simulink model "pid_and_statefeedback"  (R2021b)
settings: Solver=VariableStepAuto  StartTime=0.0  StopTime=10.0  RelTol=1e-3
undefined symbols (not defined in the file): mA, mB, mC, mD, mK, mL
libraries: slpidlib x1, simulink x1
settings Model: Creator=insha  LastModifiedBy=insha

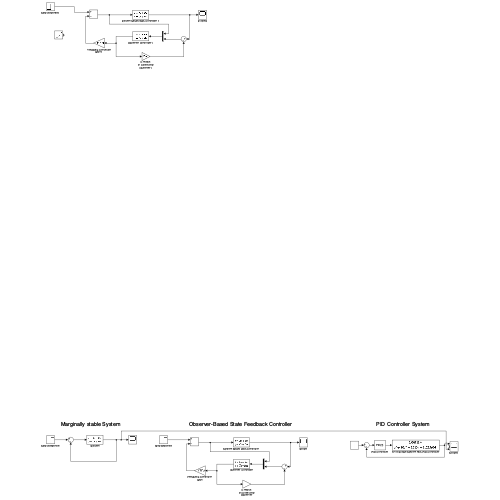
[thumbnail: Simulink's stored preview of the top-level diagram]
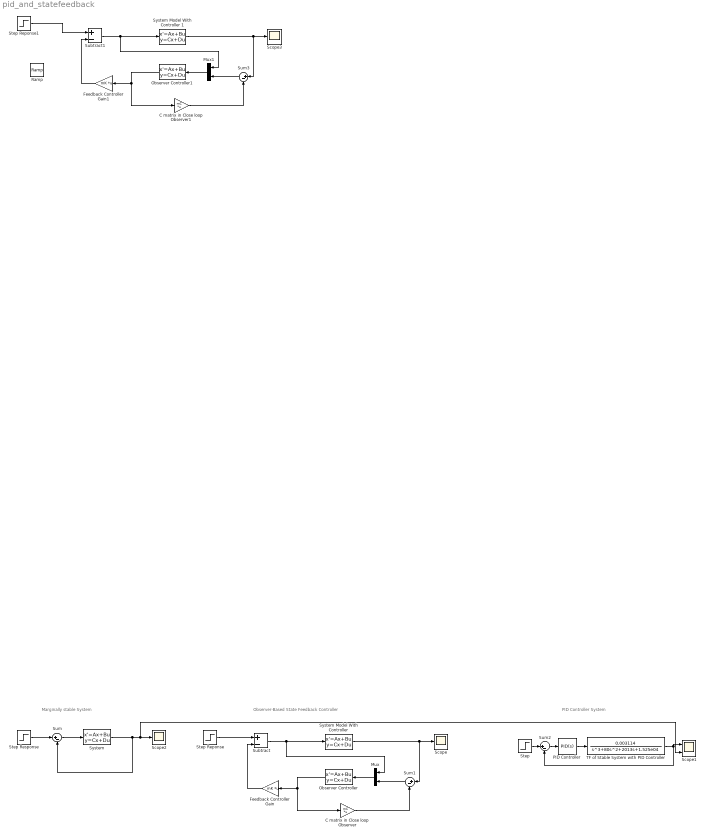
== system pid_and_statefeedback ==
  note: PID Controller System
  note: Marginally stable System
  note: Observer-Based State Feedback Controller
  " System" : StateSpace  A=mA  B=mB  C=mC  D=mD  InitialCondition=0
  C matrix in Close loop Observer : Gain  Gain=mC  Multiplication=Matrix(K*u)
  C matrix in Close loop Observer1 : Gain  Gain=mC  Multiplication=Matrix(K*u)
  Feedback Controller Gain : Gain  Gain=mK  Multiplication=Matrix(K*u)
  Feedback Controller Gain1 : Gain  Gain=mK  Multiplication=Matrix(K*u)
  Mux : Mux  Inputs=2
  Mux1 : Mux  Inputs=2
  Observer Controller : StateSpace  A=mA  B=[mB mL]  C=[1 0 0; 0 1 0; 0 0 1]  D=[0 0;0 0;0 0]  InitialCondition=0
  Observer Controller1 : StateSpace  A=mA  B=[mB mL]  C=[1 0 0; 0 1 0; 0 0 1]  D=[0 0;0 0;0 0]  InitialCondition=0
  PID Controller : slpidlib/PID Controller  Controller=PID  Form=Parallel  TimeDomain=Continuous-time  UseExternalTs=off  SampleTime=-1  IntegratorMethod=Forward Euler  FilterMethod=Forward Euler  ControllerParametersSource=internal  P=10599414.9219599  I=83189948.7980299  D=335136.517629795  UseFilter=on  N=2140.45218900231  TunerSelectOption=Transfer Function Based (PID Tuner App)  InitialConditionSource=internal  InitialConditionForIntegrator=0  InitialConditionForFilter=0  DifferentiatorICPrevScaledInput=0  ExternalReset=none  TrackingMode=off  Kt=1  LimitOutput=off  SatLimitsSource=internal  UpperSaturationLimit=inf  LowerSaturationLimit=-inf  LinearizeAsGain=on  AntiWindupMode=none  Kb=1  POutMin=[]  POutMax=[]  IOutMin=[]  IOutMax=[]  DOutMin=[]  DOutMax=[]  NOutMin=[]  NOutMax=[]  SumOutMin=[]  SumOutMax=[]  SaturationOutMin=[]  SaturationOutMax=[]  PParamMin=[]  PParamMax=[]  IParamMin=[]  IParamMax=[]  DParamMin=[]  DParamMax=[]  NParamMin=[]  NParamMax=[]  KbParamMin=[]  KbParamMax=[]  KtParamMin=[]  KtParamMax=[]  KbOutMin=[]  KbOutMax=[]  KtOutMin=[]  KtOutMax=[]  IntegratorOutMin=[]  IntegratorOutMax=[]  FilterOutMin=[]  FilterOutMax=[]  SumI1OutMin=[]  SumI1OutMax=[]  SumI2OutMin=[]  SumI2OutMax=[]  SumI3OutMin=[]  SumI3OutMax=[]  SumI4OutMin=[]  SumI4OutMax=[]  SumDOutMin=[]  SumDOutMax=[]  DifferentiatorOutMin=[]  DifferentiatorOutMax=[]  FilterDiffOutCoefMin=[]  FilterDiffOutCoefMax=[]  ReciprocalOutMin=[]  ReciprocalOutMax=[]  SumDenOutMin=[]  SumDenOutMax=[]  SumNumOutMin=[]  SumNumOutMax=[]  DivideOutMin=[]  DivideOutMax=[]  UdiffTsProdOutMin=[]  UdiffTsProdOutMax=[]  NTsProdOutMin=[]  NTsProdOutMax=[]  UintegralTsProdOutMin=[]  UintegralTsProdOutMax=[]  UngainTsProdOutMin=[]  UngainTsProdOutMax=[]  IntegratorContinuousStateAttributes=''  IntegratorStateMustResolveToSignalObject=off  IntegratorRTWStateStorageClass=Auto  FilterContinuousStateAttributes=''  FilterStateMustResolveToSignalObject=off  FilterRTWStateStorageClass=Auto  ParallelPVariant=InternalParameters  IdealPVariant=Disabled  IVariant=InternalParameters  DVariant=InternalParameters  IntegratorVariant=Continuous  SatVariant=Disabled  AWVariant=Passthrough  PCopyVariant=Disabled  TRVariant=Disabled  FdbkBlocksVariant=Forward  IdealPFdbkVariant=Disabled  SatFdbkVariant=Disabled  DerivativeFilterVariant=ContFilter  NVariant=InternalParameters  NCopyVariant=Disabled  FilterICVariant=InternalICsFilter  IntegratorICVariant=InternalICs  ExternalResetVariant=Disabled  TRSumVariant=Passthrough  SumFdbkVariant=Disabled  SumVariant=Sum_PID  TsampFilterVariant=InternalTs  TsampNgainVariant=Passthrough  TsampIntegralVariant=Passthrough  ExternalSaturationOutDataTypeStr=Inherit: Same as second input
  Ramp : simulink/Sources/Ramp  slope=5  start=0  InitialOutput=0
  Scope : Scope
  Scope1 : Scope  NumInputPorts=3
  Scope2 : Scope
  Scope3 : Scope
  Step : Step  SampleTime=0
  Step Reponse : Step  SampleTime=0
  Step Reponse1 : Step  After=5  SampleTime=0
  Step Response : Step  SampleTime=0
  Subtract : Sum  Inputs=+-
  Subtract1 : Sum  Inputs=+-
  Sum{,1..3} (4 alike) : Sum  Inputs=|+-
  "System Model With Controller " : StateSpace  A=mA  B=mB  C=mC  D=mD  InitialCondition=0
  System Model With Controller 1 : StateSpace  A=mA  B=mB  C=mC  D=mD  InitialCondition=0
  TF of Stable System with PID Controller : TransferFcn  Numerator=[0.003114]  Denominator=[1 80 2013 1.525e04]
  wires:
  "System Model With Controller "/1 -> Sum1/1, Scope/1
  Step Reponse/1 -> Subtract/1
  Subtract/1 -> Mux/1, "System Model With Controller "/1
  C matrix in Close loop Observer/1 -> Sum1/2
  Mux/1 -> Observer Controller/1
  Observer Controller/1 -> C matrix in Close loop Observer/1, Feedback Controller Gain/1
  Feedback Controller Gain/1 -> Subtract/2
  Sum1/1 -> Mux/2
  Step Response/1 -> Sum/1
  Sum/1 -> " System"/1
  " System"/1 -> Scope1/3, Scope2/1, Sum/2
  TF of Stable System with PID Controller/1 -> Sum2/2, Scope1/1
  Step/1 -> Sum2/1
  Sum2/1 -> PID Controller/1
  PID Controller/1 -> TF of Stable System with PID Controller/1
  Feedback Controller Gain1/1 -> Subtract1/2
  Subtract1/1 -> Mux1/1, System Model With Controller 1/1
  C matrix in Close loop Observer1/1 -> Sum3/2
  System Model With Controller 1/1 -> Sum3/1, Scope3/1
  Observer Controller1/1 -> C matrix in Close loop Observer1/1, Feedback Controller Gain1/1
  Sum3/1 -> Mux1/2
  Mux1/1 -> Observer Controller1/1
  Step Reponse1/1 -> Subtract1/1
